simulink model "p10"  (R2021b)
settings: Solver=VariableStepAuto  StartTime=0.0  StopTime=1e4  MaxStep=0.01
libraries: simulink x3
settings Model: Creator=user  LastModifiedBy=user

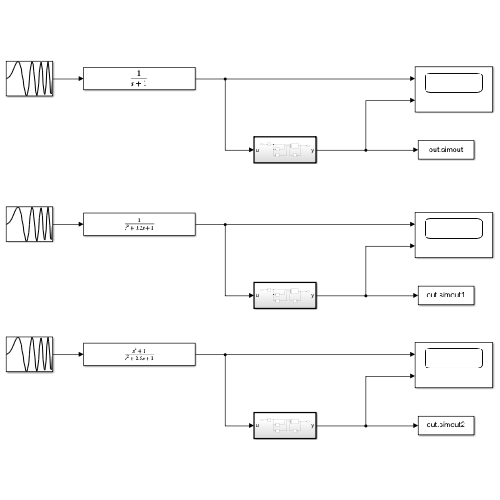
[thumbnail: Simulink's stored preview of the top-level diagram]
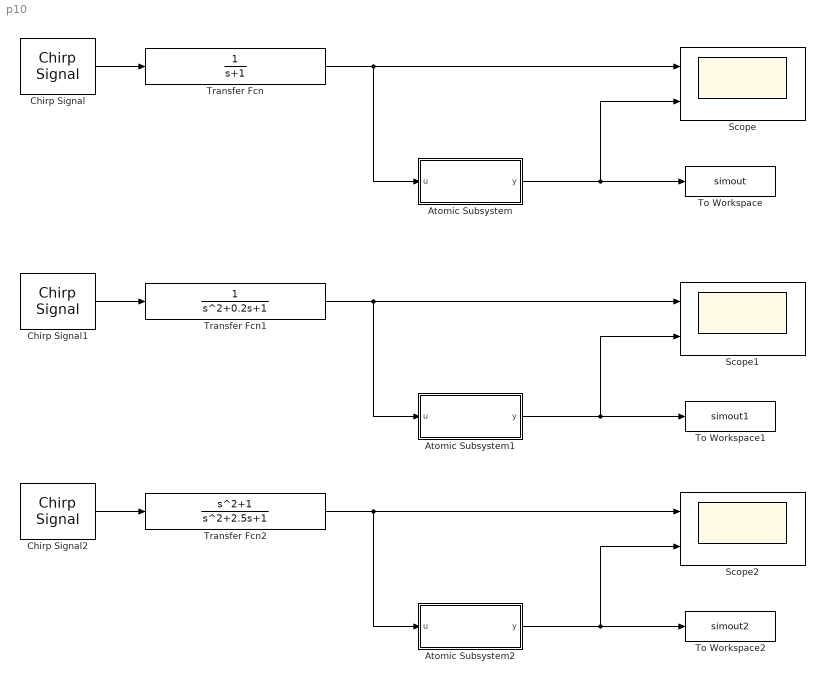
== system p10 ==
  Atomic Subsystem : Subsystem  TreatAsAtomicUnit=on
  Atomic Subsystem1 : Subsystem  TreatAsAtomicUnit=on
  Atomic Subsystem2 : Subsystem  TreatAsAtomicUnit=on
  Chirp Signal : simulink/Sources/Chirp Signal  f1=0.01/2/pi  T=1e4  f2=10/2/pi
  Chirp Signal1 : simulink/Sources/Chirp Signal  f1=0.01/2/pi  T=1e4  f2=10/2/pi
  Chirp Signal2 : simulink/Sources/Chirp Signal  f1=0.01/2/pi  T=1e4  f2=10/2/pi
  Scope : Scope  NumInputPorts=2
  Scope1 : Scope  NumInputPorts=2
  Scope2 : Scope  NumInputPorts=2
  To Workspace : ToWorkspace  VariableName=simout  SaveFormat=Timeseries  SampleTime=-1
  To Workspace1 : ToWorkspace  VariableName=simout1  SaveFormat=Timeseries  SampleTime=-1
  To Workspace2 : ToWorkspace  VariableName=simout2  SaveFormat=Timeseries  SampleTime=-1
  Transfer Fcn : TransferFcn  Numerator=[1 ]  Denominator="[1  1]"
  Transfer Fcn1 : TransferFcn  Denominator=[1 0.2 1]
  Transfer Fcn2 : TransferFcn  Numerator=[1 0 1]  Denominator=[1 2.5 1]
  wires:
  Chirp Signal/1 -> Transfer Fcn/1
  Transfer Fcn/1 -> Scope/1, Atomic Subsystem/1(u)
  Atomic Subsystem/1(y) -> To Workspace/1, Scope/2
  Transfer Fcn1/1 -> Scope1/1, Atomic Subsystem1/1(u)
  Chirp Signal1/1 -> Transfer Fcn1/1
  Atomic Subsystem1/1(y) -> To Workspace1/1, Scope1/2
  Transfer Fcn2/1 -> Scope2/1, Atomic Subsystem2/1(u)
  Chirp Signal2/1 -> Transfer Fcn2/1
  Atomic Subsystem2/1(y) -> To Workspace2/1, Scope2/2

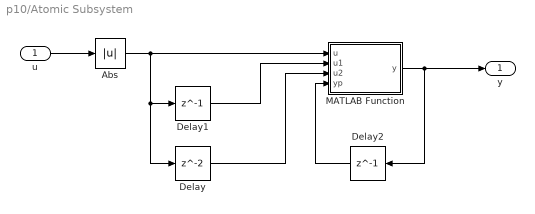
== system p10/Atomic Subsystem ==
  u : Inport
  Abs : Abs
  Delay : Delay
  Delay1 : Delay  DelayLength=1
  Delay2 : Delay  DelayLength=1  InitialCondition=1
  MATLAB Function : MATLAB Function  TreatAsAtomicUnit=on
  y : Outport
  wires:
  u/1 -> Abs/1
  Abs/1 -> Delay/1, Delay1/1, MATLAB Function/1(u)
  Delay1/1 -> MATLAB Function/2(u1)
  Delay/1 -> MATLAB Function/3(u2)
  Delay2/1 -> MATLAB Function/4(yp)
  MATLAB Function/1(y) -> y/1, Delay2/1

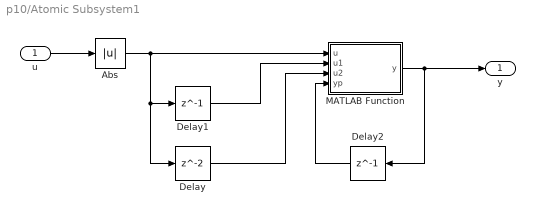
== system p10/Atomic Subsystem1 ==
  u : Inport
  Abs : Abs
  Delay : Delay
  Delay1 : Delay  DelayLength=1
  Delay2 : Delay  DelayLength=1  InitialCondition=1
  MATLAB Function : MATLAB Function  TreatAsAtomicUnit=on
  y : Outport
  wires:
  u/1 -> Abs/1
  Abs/1 -> Delay/1, Delay1/1, MATLAB Function/1(u)
  Delay1/1 -> MATLAB Function/2(u1)
  Delay/1 -> MATLAB Function/3(u2)
  Delay2/1 -> MATLAB Function/4(yp)
  MATLAB Function/1(y) -> y/1, Delay2/1

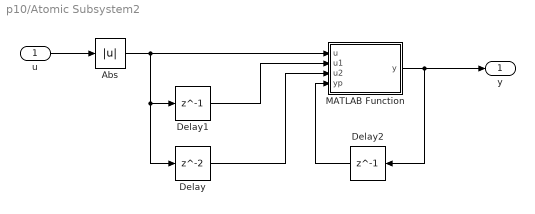
== system p10/Atomic Subsystem2 ==
  u : Inport
  Abs : Abs
  Delay : Delay
  Delay1 : Delay  DelayLength=1
  Delay2 : Delay  DelayLength=1  InitialCondition=1
  MATLAB Function : MATLAB Function  TreatAsAtomicUnit=on
  y : Outport
  wires:
  u/1 -> Abs/1
  Abs/1 -> Delay/1, Delay1/1, MATLAB Function/1(u)
  Delay1/1 -> MATLAB Function/2(u1)
  Delay/1 -> MATLAB Function/3(u2)
  Delay2/1 -> MATLAB Function/4(yp)
  MATLAB Function/1(y) -> y/1, Delay2/1

== matlab function p10/Atomic Subsystem1/MATLAB Function ==
  data: u input; y output; u1 input; u2 input; yp input
function y = fcn(u,u1,u2,yp)

    if((u1>u2)&&(u1>u))
            y = u;

    else
        y =yp;
    end

== matlab function p10/Atomic Subsystem/MATLAB Function ==
  data: u input; y output; u1 input; u2 input; yp input
function y = fcn(u,u1,u2,yp)

    if((u1>u2)&&(u1>u))
            y = u;

    else
        y =yp;
    end

== matlab function p10/Atomic Subsystem2/MATLAB Function ==
  data: u input; y output; u1 input; u2 input; yp input
function y = fcn(u,u1,u2,yp)

    if((u1>u2)&&(u1>u))
            y = u;

    else
        y =yp;
    end
